simulink model "EulerPIDJoint"  (Simulink 7.6)
settings: Solver=ode15s  StartTime=0.0  StopTime=8  FixedStep=Ts  RelTol=1e-3
InitFcn:
  | eval('Config');
  | eval('RobotCtlCfg');
values from neighbouring files (symbols this model uses):
  a2 = 0    [Config.m]    (also in CtrPlatformCfg.m)
  a3 = 0    [Config.m]    (also in CtrPlatformCfg.m)
  a4 = 0    [Config.m]    (also in CtrPlatformCfg.m)
  a5 = 90    [Config.m]    (also in CtrPlatformCfg.m)
  a6 = 0    [Config.m]    (also in CtrPlatformCfg.m)
  Cen_EU = Cen    [DynEulerTest.m]
  DH_EU = [266     300     0       0       1016     0      174 ... (first row only)    [DynEulerTest.m]
  freq = tvel/radius    (= 1)    [Config.m]    (also in CtrPlatformCfg.m)
  Ft_EU = [0;0;0;0;0;0]    [DynEulerTest.m]
  Gravity = 9.8    [Config.m]    (also in CtrPlatformCfg.m)
  Ie_EU = [Ie1;Ie2;Ie3;Ie4;Ie5;Ie6]    [DynEulerTest.m]
  in1 = [5.2954 -0.2565 -0.6366;-0.2565 4.7000 0.2830;-0.6366 0.2829 5.8635]    [Config.m]    (also in CtrPlatformCfg.m; DynEulerTest.m; EfDynCAD.m = [0.54  -0.01 0.23)
  in2 = [5.8840 0.0072 0.0135;0.0072 6.0178 -0.1907;0.0135 -0.1907 0.3374]    [Config.m]    (also in CtrPlatformCfg.m; DynEulerTest.m; EfDynCAD.m = (R_x*R_z)*in2*(R_x*R_z)')
  in3 = [1.8201 -0.2274 -0.3112;-0.2274 2.2537 -0.1441;-0.3112 -0.1441 1.9485]    [Config.m]    (also in CtrPlatformCfg.m; DynEulerTest.m; EfDynCAD.m = (R_x*R_z)*in3*(R_x*R_z)')
  in4 = [0.0607 -0.0922 0;-0.0922 1.4493 0;0 0 1.4620]    [Config.m]    (also in CtrPlatformCfg.m; DynEulerTest.m = [0.0607 -0.0922 0;-0.0922 1.4493 0;0 0,1.4620]; EfDynCAD.m = (R_y*Rz)*in4*(R_y*Rz)')
  in5 = [0.0191 0.0032 0;0.0032 0.0228 0;0 0 0.0291]    [Config.m]    (also in CtrPlatformCfg.m; DynEulerTest.m; EfDynCAD.m = (R_x*R_y)*in5*(R_x*R_y)')
  in6 = [0.0012 0 0;0 0.0007 0;0 0 0.0007]    [Config.m]    (also in CtrPlatformCfg.m; DynEulerTest.m; EfDynCAD.m = (R_y*Rz)*in6*(R_y*Rz)')
  init_Endx = gd_init(1,4)    [Config.m]    (also in CtrPlatformCfg.m)
  init_Endy = gd_init(2,4)    [Config.m]    (also in CtrPlatformCfg.m)
  init_Endz = gd_init(3,4)    [Config.m]    (also in CtrPlatformCfg.m)
  init_Rot = gd_init(1:3,1:3)    [Config.m]    (also in CtrPlatformCfg.m)
  L = [l1 l2 l3 l4 l5 l6 l7 l8 l9]    [Config.m]    (also in CtrPlatformCfg.m)
  ma1 = 170.31    [Config.m]    (also in CtrPlatformCfg.m; DynEulerTest.m; EfDynCAD.m = 77.75)
  ma2 = 63.74    [Config.m]    (also in CtrPlatformCfg.m; DynEulerTest.m; EfDynCAD.m = 32.31)
  ma3 = 98.98    [Config.m]    (also in CtrPlatformCfg.m; DynEulerTest.m; EfDynCAD.m = 18.61)
  ma4 = 24.46    [Config.m]    (also in CtrPlatformCfg.m; DynEulerTest.m; EfDynCAD.m = 15.65)
  ma5 = 5.24    [Config.m]    (also in CtrPlatformCfg.m; DynEulerTest.m; EfDynCAD.m = 3.32)
  ma6 = 0.6    [Config.m]    (also in CtrPlatformCfg.m; DynEulerTest.m; EfDynCAD.m)
  Ma_EU = Ma    [DynEulerTest.m]
  tvel = 120    [Config.m]    (also in CtrPlatformCfg.m)
undefined symbols (not defined in the file or in its folder): a1, jointAugKp, jointAugKv
libraries: mblibv1 x41, simulink x5
(part 4 of 4)

== matlab function Feedforward/Newton Euler Recursion ==
  data: RefPos input double; Torque output double; RefVel input double; RefAcc input double; EnPos input double; EnVel input double; EnAcc input double; DH_EU parameter double; Ma_EU parameter double; Cen_EU parameter double; Ie_EU parameter double; Ft_EU parameter double; JntVel output double; JntAcc output double; JntF output double
function [Torque,JntVel,JntAcc,JntF]= fcn(RefPos,RefVel,RefAcc,EnPos,EnVel,EnAcc,DH_EU,Ma_EU,Cen_EU,Ie_EU,Ft_EU)
%#eml
JntVel=zeros(36,1);
JntAcc=zeros(36,1);
JntF=zeros(36,1);
Torque = [0;0;0;0;0;0];
%%%%%%%%%%Make use of encoder feedback information%%%%%%%%%%%%%
[Torque,JntVel,JntAcc,JntF] = DynEulerCon(DH_EU,Ma_EU,Cen_EU,Ie_EU,Ft_EU,RefPos,RefVel,RefAcc,EnPos,EnVel,EnAcc);
%%%%%%%%%%Not use encoder feedback information%%%%%%%%%%%%%%%%%
%[Torque,JntVel,JntAcc,JntF] = DynEuler(DH_EU,Ma_EU,Cen_EU,Ie_EU,Ft_EU,RefPos,RefVel,RefAcc);

== matlab function Trajectory Generator/Circle in Descartes Space/Inverse Kinematic ==
  data: EndPos input double; init_Rot parameter double; Theta output double; L parameter double
function Theta = fcn(EndPos,init_Rot,L)
%#eml
Theta =[0;0; 0; 0; 0; 0];
gd = [init_Rot,EndPos;[0 0 0],1];
[Theta_total,num_total] = inv_kin(gd,L);
%%%%%%%%%%%Need to modify%%%%%%%%%%%%%%%
Theta = Theta_total(:,2);

== matlab function Trajectory Generator/Circle in Descartes Space/Jacobian ==
  data: Theta input double; Omega output double; EndVel input double; L parameter double
function Omega = fcn(Theta,EndVel,L)
%#eml

Omega = zeros(6,1);
V = [EndVel; 0; 0; 0];   
g = fwd_kin(L,Theta');
Jb = body_Jacobian(L,Theta');
Adg_inv = double(AdjointInv(g));
Omega = double((Jb \ Adg_inv* V)')';

== matlab function Trajectory Generator/Line in Joint Space/Forward ==
  data: Theta input double; EndPos output double; L parameter double
function EndPos = fcn(Theta,L)
%#eml
gd = fwd_kin(L,Theta');
EndPos = gd(1:3,4);

== matlab function Trajectory Generator/Line in Joint Space/Jacobian ==
  data: Theta input double; Omega input double; EndVel output double; L parameter double
function EndVel = fcn(Theta,Omega,L)
%#eml


EndVW = spat_Jacobian(L,Theta')*Omega;
gd = fwd_kin(L,Theta');
EndW = EndVW(4:6,1);
gd_pos = gd(1:3,4);
EndVel=cross(EndW,gd_pos);
